simulink model "fully_controlled_bridgle_rectifier"  (R2022a)
settings: Solver=VariableStepAuto  StartTime=0.0  StopTime=0.04  RelTol=1e-3
libraries: spsThyristorLib x4, spsVoltageMeasurementLib x3, spsACVoltageSourceLib x1, spsCurrentMeasurementLib x1, spsGroundLib x1, spsParallelRLCBranchLib x1, spspowerguiLib x1
settings Model: Creator=P.O.M.G  LastModifiedBy=P.O.M.G

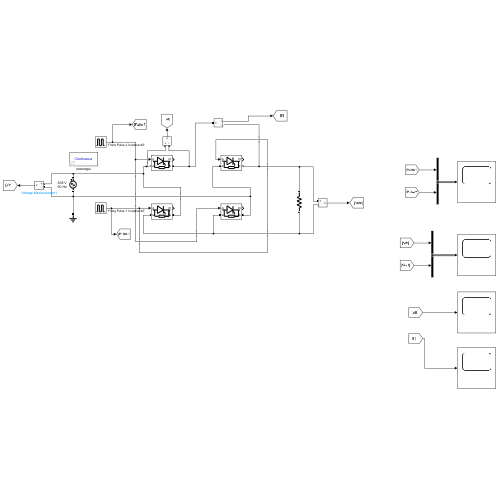
[thumbnail: Simulink's stored preview of the top-level diagram]
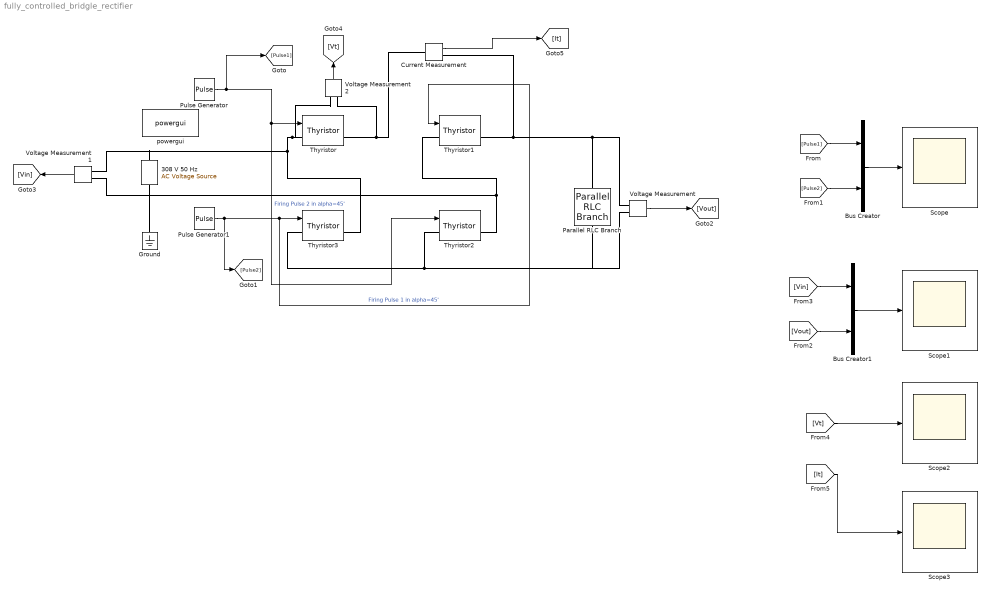
== system fully_controlled_bridgle_rectifier ==
  308 V 50 Hz : spsACVoltageSourceLib/AC Voltage Source  Amplitude=308  Phase=0  Frequency=50  SampleTime=0  Measurements=None  BusType=swing  Pref=10e3  Qref=0  Qmin=-inf  Qmax=+inf
  Bus Creator : BusCreator  Inputs=2
  Bus Creator1 : BusCreator  Inputs=2
  Current Measurement : spsCurrentMeasurementLib/Current Measurement  PhasorSimulation=off  OutputType=Complex  PSBequivalent=0
  Ground : spsGroundLib/Ground  LConnTagsString=a
  Parallel RLC Branch : spsParallelRLCBranchLib/Parallel RLC Branch  LConnTagsString=a  RConnTagsString=__new0  BranchType=R  Resistance=100  Inductance=1e-3  SetiL0=off  InitialCurrent=0  Capacitance=1e-6  Setx0=off  InitialVoltage=0  Measurements=None
  Pulse Generator : DiscretePulseGenerator  PulseType=Time based  Period=0.02  PulseWidth=5  PhaseDelay=.0025
  Pulse Generator1 : DiscretePulseGenerator  PulseType=Time based  Period=0.02  PulseWidth=5  PhaseDelay=0.05
  Scope{,1..3} (4 alike) : Scope
  Thyristor{,1..3} (4 alike) : spsThyristorLib/Thyristor  Ron=0.001  Lon=0  Vf=0.8  IC=0  Rs=500  Cs=250e-9  Measurements=on
  Voltage Measurement : spsVoltageMeasurementLib/Voltage Measurement  PhasorSimulation=off  OutputType=Complex  PSBequivalent=0
  Voltage Measurement1 : spsVoltageMeasurementLib/Voltage Measurement  PhasorSimulation=off  OutputType=Complex  PSBequivalent=0
  Voltage Measurement2 : spsVoltageMeasurementLib/Voltage Measurement  PhasorSimulation=off  OutputType=Complex  PSBequivalent=0
  powergui : spspowerguiLib/powergui  Priority=1  SimulationMode=Continuous  SampleTime=50e-6  frequency=60  Iterations=50  frequencyindice=50  Pbase=100e6  ErrMax=1e-4  UnitsV=kV  UnitsW=MW  buscounter=0  FunctionMessages=off  echomessages=off  EnableUseOfTLC=off  CurrentSourceSwitches=off  DisableSnubberDevices=off  DisableRonSwitches=off  DisableVfSwitches=off  DisplayEquations=off  AutomaticDiscreteSolvers=off  SolverType=Tustin/Backward Euler (TBE)  Interpol=off  ExternalGateDelay=off  methode=off  Ts=100  x0status=blocks  SPID=on  SwTol=0  HookPort=off  NonlinearTolerance=1e-4  nMaxIteration=100  ContinueOnMaxIteration=off  RestoreLinks=warning  ResistiveCurrentMeasurement=off  Frange=[0:2:500]  Ylog=off  Xlog=on  ShowGrid=off  save=off  variable=ZData  structure=0  ZoomFFT=off  StartTime=0.0  cycles=1  DisplayStyle=1  fundamental=60  FreqAxis=off  MaxFrequency=1000  frequencyindicesteady=1  RmsSteady=1  display=off
  wires:
  Pulse Generator/1 -> [Pulse1], Thyristor2/1, Thyristor/1  "Firing Pulse 2 in alpha=45'"
  Pulse Generator1/1 -> [Pulse2], Thyristor3/1, Thyristor1/1  "Firing Pulse 1 in alpha=45'"
  Bus Creator/1 -> Scope/1
  [Pulse1] -> Bus Creator/1
  [Pulse2] -> Bus Creator/2
  Voltage Measurement/1 -> [Vout]
  Voltage Measurement1/1 -> [Vin]
  Voltage Measurement2/1 -> [Vt]
  [It] -> Scope3/1
  [Vt] -> Scope2/1
  Current Measurement/1 -> [It]
  Bus Creator1/1 -> Scope1/1
  [Vin] -> Bus Creator1/1
  [Vout] -> Bus Creator1/2
  connections:
  Thyristor3/RConn1 -- 308 V 50 Hz/RConn1 -- Voltage Measurement1/LConn1 -- Voltage Measurement2/LConn1 -- Thyristor/LConn1
  Thyristor2/RConn1 -- Voltage Measurement1/LConn2 -- 308 V 50 Hz/LConn1 -- Ground/LConn1 -- Thyristor1/LConn1
  Thyristor3/LConn1 -- Parallel RLC Branch/RConn1 -- Voltage Measurement/LConn2 -- Thyristor2/LConn1
  Thyristor1/RConn1 -- Current Measurement/RConn1 -- Voltage Measurement/LConn1 -- Parallel RLC Branch/LConn1
  Thyristor/RConn1 -- Voltage Measurement2/LConn2 -- Current Measurement/LConn1
